simulink model "demo2"  (Simulink 7.1)
settings: Solver=ode45  StartTime=0.0  StopTime=10.0  RelTol=1e-3
libraries: roblocks x2, simulink x1
settings Model: Creator=pic  LastModifiedBy=pic  ExtModeTrigMode=oneshot  ExtModeArmWhenConnect=off
settings DataIOCC: LimitDataPoints=off
settings OptimizationCC: BlockReduction=off  BooleanDataType=off
settings DebuggingCC: SaveWithParameterizedLinksMsg=none  SignalResolutionControl=TryResolveAllWithWarning  SolverPrmCheckMsg=none  MultiTaskDSMMsg=warning  MultiTaskCondExecSysMsg=none  StrictBusMsg=None
settings HardwareCC: TargetUnknown=on
settings RTWCC: IncludeERTFirstTime=on
settings GRTTargetCC: ModelReferenceCompliant=off  CompOptLevelCompliant=off  MatFileLogging=off

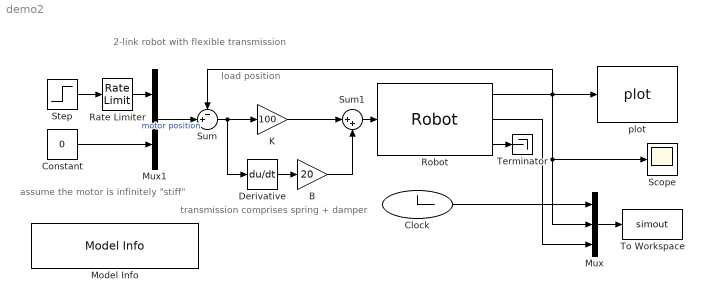
== system demo2 ==
  note: 2-link robot with flexible transmission
  note: load position
  note: transmission comprises
      | spring + damper
  note: assume the motor
      | is infinitely "stiff"
  B : Gain  Gain=20  SaturateOnIntegerOverflow=on  OutDataTypeStr=Inherit: Same as input  ParamDataTypeStr=Inherit: Same as input
  Clock : Clock
      settings: Decimation=10
  Constant : Constant  Value=0
  Derivative : Derivative
  K : Gain  Gain=100  SaturateOnIntegerOverflow=on  OutDataTypeStr=Inherit: Same as input  ParamDataTypeStr=Inherit: Same as input
  Model Info : simulink/Model-Wide Utilities/Model Info  SystemSampleTime=-1  InitialBlockCM=none  BlockCM=none  Frame=on  DisplayStringWithTags=|  HorizontalTextAlignment=Left  LeftAlignmentValue=0.02  SourceBlockDiagram=demo2  TagMaxNumber=20
      | 2-link demo
      | %<Creator>
      | %<ModifiedDate>
  Mux : Mux  Inputs=3
  Mux1 : Mux  Inputs=2
  Rate Limiter : RateLimiter  RisingSlewLimit=50  FallingSlewLimit=-50
  Robot : roblocks/Robot  SystemSampleTime=-1  robot=tl  q0=[0 0]
  Scope : Scope
      settings: YMin=-0.5  YMax=1.5
  Step : Step  SampleTime=0
  Sum : Sum  Inputs=-+|  SaturateOnIntegerOverflow=on  InputSameDT=on  OutDataTypeStr=Inherit: Same as first input
  Sum1 : Sum  Inputs=|++  SaturateOnIntegerOverflow=on  InputSameDT=on  OutDataTypeStr=Inherit: Same as first input
  Terminator : Terminator
  To Workspace : ToWorkspace  VariableName=simout  SampleTime=-1  SaveFormat=Array
  plot : roblocks/plot  SystemSampleTime=-1  robot=tl
  wires:
  Constant/1 -> Mux1/2
  Step/1 -> Rate Limiter/1
  Rate Limiter/1 -> Mux1/1
  Sum/1 -> K/1, Derivative/1
  Robot/1 -> plot/1, Sum/1, Mux/2, Scope/1
  Sum1/1 -> Robot/1
  K/1 -> Sum1/1
  B/1 -> Sum1/2
  Derivative/1 -> B/1
  Mux1/1 -> Sum/2  "motor position"
  Mux/1 -> To Workspace/1
  Clock/1 -> Mux/1
  Robot/2 -> Mux/3
  Robot/3 -> Terminator/1
